simulink model "TDPBehaviourSim"  (R2020b)
settings: Solver=VariableStepAuto  StartTime=0.0  StopTime=200  FixedStep=sampleTime  RelTol=1e-3  EnableMultiTasking=on
values from neighbouring files (symbols this model uses):
  angThresh = pi/16    (= 0.196349540849)    [GameParameters.m]
  attackerKickSpeed = 0.3    [GameParameters.m]
  AwayFormation1 = [9.5 4 pi ... (first row only)    [FormationPoses.m]    (also in GameParameters.m)
  ballAngleNoise = pi/24    (= 0.1308996939)    [GameParameters.m]
  ballThresh = playerRadius + 0.03    (= 0.11)    [GameParameters.m]
  ballVelNoise = 0.05    [GameParameters.m]
  distThresh = 0.1    [GameParameters.m]
  fieldCenter = [mean(fieldLimitsX) mean(fieldLimitsY)]    [GameParameters.m]
  fieldLimitsX = [1 10]    [GameParameters.m]
  fieldLimitsY = [1 7]    [GameParameters.m]
  goalPosts = [1  2.7 2 ... (first row only)    [GameParameters.m]
  HomeFormation1 = [1.5 4 0 ... (first row only)    [FormationPoses.m]    (also in GameParameters.m)
  maxSpeed = 0.1    [GameParameters.m]
  maxTurnSpeed = 0.05    [GameParameters.m]
  playerRadius = 0.08    [GameParameters.m]
  sampleTime = 0.5    [GameParameters.m]
undefined symbols (not defined in the file or in its folder): DiscIntNeverNeededParam
libraries: mobileRoboticsLib x33, soccerRobotLib x16
(part 2 of 2)

== system TDPBehaviourSim/Home Team/GK Information for Decision Making ==
  In1 : Inport
  In2 : Inport  Port=2
  Personal Information : BusSelector  OutputSignals=Home Team GK pos,Home Team GK obj,Home Team GK robot,Home GK Velocity
  TeamMatePositions : BusSelector  OutputSignals=Home Team Defender pos,Home Team MidFielder pos,Home Team Striker pos
  <Home Team GK pos> : Outport
  <Home Team GK obj> : Outport  Port=2
  <Home Team GK robot> : Outport  Port=3
  <Home GK Velocity> : Outport  Port=4
  <Home Team Defender pos> : Outport  Port=5
  <Home Team MidFielder pos> : Outport  Port=6
  <Home Team Striker pos> : Outport  Port=7
  wires:
  Personal Information/2 -> <Home Team GK obj>/1  "<Home Team GK obj>"
  Personal Information/4 -> <Home GK Velocity>/1  "<Home GK Velocity>"
  TeamMatePositions/3 -> <Home Team Striker pos>/1  "<Home Team Striker pos>"
  In1/1 -> Personal Information/1
  In2/1 -> TeamMatePositions/1
  Personal Information/1 -> <Home Team GK pos>/1  "<Home Team GK pos>"
  TeamMatePositions/1 -> <Home Team Defender pos>/1  "<Home Team Defender pos>"
  Personal Information/3 -> <Home Team GK robot>/1  "<Home Team GK robot>"
  TeamMatePositions/2 -> <Home Team MidFielder pos>/1  "<Home Team MidFielder pos>"

== system TDPBehaviourSim/Home Team/MidFielder Information For Decision Making ==
  In1 : Inport
  In2 : Inport  Port=2
  Bus Selector : BusSelector  OutputSignals=Home Team Midfielder obj,Home Team Midfielder robot,Home Team MidFielder pos,Home Mid Vel
  Bus Selector1 : BusSelector  OutputSignals=Home Team Striker pos,Home Team Defender pos,Home Team GK pos
  <Home Team Midfielder obj> : Outport
  <Home Team Midfielder robot> : Outport  Port=2
  <Home Team MidFielder pos> : Outport  Port=3
  <Home Mid Vel> : Outport  Port=4
  <Home Team Striker pos> : Outport  Port=5
  <Home Team Defender pos> : Outport  Port=6
  <Home Team GK pos> : Outport  Port=7
  wires:
  Bus Selector1/3 -> <Home Team GK pos>/1  "<Home Team GK pos>"
  Bus Selector1/1 -> <Home Team Striker pos>/1  "<Home Team Striker pos>"
  Bus Selector/1 -> <Home Team Midfielder obj>/1  "<Home Team Midfielder obj>"
  In2/1 -> Bus Selector/1
  In1/1 -> Bus Selector1/1
  Bus Selector1/2 -> <Home Team Defender pos>/1  "<Home Team Defender pos>"
  Bus Selector/2 -> <Home Team Midfielder robot>/1  "<Home Team Midfielder robot>"
  Bus Selector/3 -> <Home Team MidFielder pos>/1  "<Home Team MidFielder pos>"
  Bus Selector/4 -> <Home Mid Vel>/1  "<Home Mid Vel>"

== system TDPBehaviourSim/Home Team/Striker Information fot Decision Making ==
  In1 : Inport
  In2 : Inport  Port=2
  Bus Selector : BusSelector  OutputSignals=Home Team Striker robot,Home Team Striker obj,Home Team Striker pos,Home Striker Vel
  Bus Selector1 : BusSelector  OutputSignals=Home Team GK pos,Home Team Defender pos,Home Team MidFielder pos
  <Home Team Striker robot> : Outport
  <Home Team Striker obj> : Outport  Port=2
  <Home Team Striker pos> : Outport  Port=3
  <Home Striker Vel> : Outport  Port=4
  <Home Team GK pos> : Outport  Port=5
  <Home Team Defender pos> : Outport  Port=6
  <Home Team MidFielder pos> : Outport  Port=7
  wires:
  Bus Selector1/1 -> <Home Team GK pos>/1  "<Home Team GK pos>"
  In1/1 -> Bus Selector/1
  In2/1 -> Bus Selector1/1
  Bus Selector/1 -> <Home Team Striker robot>/1  "<Home Team Striker robot>"
  Bus Selector/4 -> <Home Striker Vel>/1  "<Home Striker Vel>"
  Bus Selector/2 -> <Home Team Striker obj>/1  "<Home Team Striker obj>"
  Bus Selector/3 -> <Home Team Striker pos>/1  "<Home Team Striker pos>"
  Bus Selector1/3 -> <Home Team MidFielder pos>/1  "<Home Team MidFielder pos>"
  Bus Selector1/2 -> <Home Team Defender pos>/1  "<Home Team Defender pos>"

== stateflow chart TDPBehaviourSim/Away Team/Chart ==
  state Information
    en,du:
    position;
    players;
    objects
    nextVelocity = [velocity(1); velocity(2); velocity(3)];
    [objSeen,objDIst,objAng] = detectObj(objects,1);
    toObj = [objSeen,objDIst,objAng];
    teammates;
  (default) -> Information
  data: position input; velocity input size=[3 1]; nextVelocity output =[0;0;0]; players input; teammates input; objects input; objAng local; objDIst local; objSeen local; toObj output

== stateflow chart TDPBehaviourSim/Away Team/Chart1 ==
  state Information
    en,du:
    position;
    nextVelocity = [velocity(1); velocity(2); velocity(3)];
    [objSeen,objDIst,objAng] = detectObj(objects,1);
    toObj = [objSeen,objDIst,objAng];
    teammates;
    players;
    objects;
  (default) -> Information
  data: position input; velocity input size=[3 1]; nextVelocity output =[0;0;0]; players input; teammates input; objects input; toObj output; objAng local; objDIst local; objSeen local

== stateflow chart TDPBehaviourSim/Away Team/Chart2 ==
  state Information
    en,du:
    position;
    nextVelocity = [velocity(1);velocity(2);velocity(3)]
    teammates;
    players;
    [objSeen,objDIst,objAng] = detectObj(objects,1);
    toObj = [objSeen,objDIst,objAng];
    objects
  (default) -> Information
  data: position input; velocity input size=[3 1]; nextVelocity output =[0;0;0]; players input; teammates input; objects input; toObj output; objAng local; objDIst local; objSeen local

== stateflow chart TDPBehaviourSim/Away Team/Chart3 ==
  state Information
    en,du:
    position;
    nextVelocity = [velocity(1);velocity(2);velocity(3)];
    teammates;
    objects;
    players;
    [objSeen,objDIst,objAng] = detectObj(objects,1);
    toObj = [objSeen,objDIst,objAng];
  (default) -> Information
  data: position input; velocity input size=[3 1]; nextVelocity output =[0;0;0]; players input; teammates input; objects input; toObj output; objAng local; objDIst local; objSeen local

== stateflow chart TDPBehaviourSim/GameState ==
  state BallDynamics [parallel]
    en:
    setBallState(fieldCenter,0,0);
    settings: executionOrder=2
    state InBounds
      en:
      randNum = randn(1,2);
      du:
      gamestate.state = getGameState;
      state BallFree
      state BallHeld
        en,du:
        ballPose = [robo_pos(3*holder_idx-2) robo_pos(3*holder_idx-1)] + ...
        (playerRadius+ballThresh)*[cos(robo_pos(3*holder_idx)) sin(robo_pos(3*holder_idx))];
      (default) -> BallFree
      BallHeld -> BallFree : after(1,sec)[ballKicked==1]{setBallState(ballPose,ballVel + ballVelNoise,robo_pos(3*holder_idx))}
      BallFree -> BallHeld : [gamestate.possession(1)~=0]
    state OutOfBounds
      en,du:
      gamestate.state = getGameState;
      setBallState(ballPose,0,0);
      if lastPossession == 1
      end
    state CornerOrGOakKick
      en,du:
      gamestate.state = getGameState;
    state GoalScored
      en,du:
      gamestate.state = getGameState;
    (default) -> InBounds
    OutOfBounds -> InBounds : [gamestate.state==gameSituation(1)]
    InBounds -> OutOfBounds [order 1] : [gamestate.state == gameSituation(2)]
    GoalScored -> InBounds : [gamestate.state==gameSituation(1)]
    InBounds -> GoalScored [order 2] : [gamestate.state==gameSituation(3)]
    CornerOrGOakKick -> InBounds : [gamestate.state==gameSituation(1)]
    InBounds -> CornerOrGOakKick [order 3] : [gamestate.state==gameSituation(4)]
  state TimeSetter [parallel]
    en,du:
    settings: executionOrder=3
    state EarlyGame
      en,du:
      time=elapsed(sec);
      gamestate.time=gameTime(1);
    state MidGame
      en,du:
      time=elapsed(sec);
      gamestate.time=gameTime(2);
    state LateGame
      en,du:
      time=elapsed(sec);
      gamestate.time=gameTime(3)
    state GameOver
      en:
      done = 1;
    (default) -> EarlyGame
    EarlyGame -> MidGame : [time==400]
    MidGame -> LateGame : [time==800]
    LateGame -> GameOver : [time==1200]
  state state = getGameState [function]
    note: Returns the game state depending on the position of the ball on the field
    (default) -> (junction 52)
    (junction 52) -> (junction 53) [order 1] : [ballPose(1) <= fieldLimitsX(1) || ballPose(1) >= fieldLimitsX(2) || ...
        |  ballPose(2) <= fieldLimitsY(1) || ballPose(2) >= fieldLimitsY(2)]
    (junction 52) -> (junction 56) [order 2] : {state = gameSituation.InPlay;}
    (junction 53) -> (junction 54)
    (junction 54) -> (junction 55) [order 1] : [ballPose(2)<=goalPosts(1,2) && ...
        | ballPose(2) >= goalPosts(2,2)]
    (junction 54) -> (junction 57) [order 2] : {state = gameSituation.OutOfPlay;}
    (junction 55) -> (junction 58) : {state = gameSituation.GoalScored;}
    (junction 57) -> (junction 56)
    (junction 58) -> (junction 57)
  state setBallState(pos,vel,theta) [function]
  state DeterminePossession [parallel]
    en,du:
    gamestate.possession = [holded,holder_idx];
    if gamestate.possession(2)>0 &&gamestate.possession(2)<=4
    gamestate.possessingTeam = 1;
    lastPossession = 1;
    elseif gamestate.possession(2)>=5
    gamestate.possessingTeam = 2;
    lastPossession = 2;
    else
    gamestate.possessingTeam = 0;
    end
    settings: executionOrder=1
  data: sf_internal_action_state_placeholder_data local double size=1 =0; state function_output; pos function_input double size=[1 2]; vel function_input double size=1; theta function_input double size=1; ballPose output =fieldCenter; attackerKickSpeed parameter; ballThresh parameter; ballDist local; playerRadius parameter double; fieldLimitsX parameter; fieldLimitsY parameter; goalPosts parameter; fieldCenter parameter; robo_pos input; gamestate output Bus: gameSituationBus; ballVel local =0.5; ballVelNoise parameter; ballAngleNoise parameter; randNum local =[0 0]; ballKicked local =0; time local; done output =0; lastPossession local =0; holded input; holder_idx input

== stateflow chart TDPBehaviourSim/TeamActivityAssignment ==
  state SetTeamActivity [parallel]
    en,du:
    settings: executionOrder=1
    state InPlay
      state Attack
        en,du:
        homeTeam.inPossession = 1;
        homeTeam.activity = teamAction(1);
        homeTeam.ballHolder = gamestate.possession(2);
        awayTeam.inPossession = 0;
        awayTeam.activity = teamAction(2);
        awayTeam.ballHolder = 0;
      state Defend
        en,du:
        homeTeam.inPossession = 0;
        homeTeam.activity = teamAction(1);
        homeTeam.ballHolder = gamestate.possession(2);
        awayTeam.inPossession = 1;
        awayTeam.activity = teamAction(2);
        awayTeam.ballHolder = 0;
      state CaptureBall
        en,du:
        homeTeam.inPossession = 0;
        homeTeam.ballHolder = 0;
        awayTeam.inPossession = 0;
        awayTeam.ballHolder = 0;
        homeTeam.activity = teamAction(3);
        awayTeam.activity = teamAction(3);
      (default) -> (junction 7)
      (junction 25) -> Attack
      (junction 26) -> (junction 25) : [gamestate.possessingTeam==1]
      (junction 7) -> Attack [order 1] : [gamestate.possessingTeam == 1]
      (junction 7) -> (junction 10) [order 2]
      Attack -> (junction 23) [order 2]
      (junction 23) -> (junction 24) : [gamestate.possessingTeam==0]
      Attack -> Defend [order 1] : [gamestate.possessingTeam==2]
      Defend -> Attack [order 1] : [gamestate.possessingTeam==1]
      (junction 10) -> Defend [order 1] : [gamestate.possessingTeam==2]
      (junction 10) -> (junction 14) [order 2]
      Defend -> CaptureBall [order 2] : [gamestate.possessingTeam==0]
      CaptureBall -> Defend [order 1] : [gamestate.possessingTeam==2]
      (junction 14) -> CaptureBall
      (junction 24) -> CaptureBall
      CaptureBall -> (junction 26) [order 2]
    state OutOfPlay
    state GoalScored
    state GoalCornerKick
    (default) -> (junction 35)
    GoalCornerKick -> InPlay : [gamestate.state==gameSituation(1)]
    (junction 35) -> InPlay [order 1]
    (junction 35) -> (junction 39) [order 2]
    InPlay -> GoalScored [order 3] : [gamestate.state==gameSituation(3)]
    InPlay -> GoalCornerKick [order 2] : [gamestate.state==gameSituation(4)]
    InPlay -> OutOfPlay [order 1] : [gamestate.state==gameSituation(2)]
    OutOfPlay -> InPlay : [gamestate.state==gameSituation(1)]
    (junction 39) -> OutOfPlay [order 1] : [gamestate.state==gameSituation(2)]
    (junction 39) -> (junction 43) [order 2]
    (junction 43) -> GoalScored [order 1] : [gamestate.state==gameSituation(3)]
    (junction 43) -> (junction 47) [order 2]
    (junction 47) -> GoalCornerKick : [gamestate.state==gameSituation(4)]
  data: gamestate input Bus: gameSituationBus; homeTeam output Bus: teamActivity; awayTeam output Bus: teamActivity

== matlab function TDPBehaviourSim/MATLAB Function ==
  data: home input; holded output; away input; indexholder output
function [holded,indexholder]=findholder(home,away)
holded=false;
holdingTeam= 0;
indexholder=0;
awayHolds=0;
homeHolds=0;
determineholder=0;
%% This function returns if ball is holded or not and the player's index if holded
homeindexholder = find(home(:,1) ~= 0 & home(:,2) < 0.3  & home(:,2) > 0  & home(:,3) > -pi/4 & home(:,3) < pi/4);
awayindexholder = find(away(:,1) ~= 0 & away(:,2) < 0.3 & away(:,2) > 0 & away(:,3) >-pi/4  & away(:,3) < pi/4);
awayHolds = ~isempty(awayindexholder);
homeHolds = ~isempty(homeindexholder);

if awayHolds || homeHolds
    holded = true;
    if homeHolds && ~awayHolds
        if size(homeindexholder,1)== 1
            indexholder = homeindexholder(1);
        else
            indexholder = homeindexholder(randi([1,size(homeindexholder,1)]));            
        end
    elseif awayHolds && ~homeHolds
        if size(homeindexholder,1)>1
            indexholder = awayindexholder(randi([1,size(awayindexholder,1)])) + 4;
        else
            indexholder = awayindexholder(1);
        end
    elseif  homeHolds && awayHolds
        determineholder = [homeindexholder;awayindexholder+4];
        indexholder = determineholder(randi([1,size(determineholder,1)]));
    end
    
end
end

== stateflow chart TDPBehaviourSim/Home Team/Chart4 ==
  state [vel,done] = goToPose(goal) [function]
    note: Tracks a position. Once reached, the robot will turn in place until a reference angle is met.
    (default) -> (junction 225) : {
        | vel = [0;0;0];
        | [goalDist,goalAng] = calcBearing(goal(1:2));
        | trackAng = angdiff(position(3),goal(3));
        | }
    (junction 225) -> (junction 226) [order 1] : % Track the position if outside the distance threshold
        | [goalDist > distThresh]
    (junction 225) -> (junction 227) [order 2] : % Else, turn in place until the angular reference is met
    (junction 226) -> (junction 234) : {vel = trackDetection(goalDist,goalAng);}
    (junction 227) -> (junction 228) [order 1] : [trackAng > angThresh]
    (junction 227) -> (junction 229) [order 2]
    (junction 228) -> (junction 233) : {vel(3) = 1;}
    (junction 229) -> (junction 230) [order 1] : [trackAng < -angThresh]
    (junction 229) -> (junction 231) [order 2]
    (junction 230) -> (junction 232) : {vel(3) = -1;}
    (junction 232) -> (junction 231)
    (junction 233) -> (junction 232)
    (junction 234) -> (junction 233)
    (junction 231) -> (junction 235) : {done = (goalDist <= distThresh) && (abs(trackAng) <= angThresh);}
  state PlayerMovement [parallel]
    en:
    nextVelocity = velocity;
    du:
    settings: executionOrder=1
    state InPlay
      state Attack
        state BallHolder
          en,du:
          nextVelocity = goToPose([1,4,0]);
        state OtherTeammateBallHolder
          en,du:
          nextVelocity=goToPose([8,3,0]);
        (default) -> (junction 338)
        (junction 338) -> BallHolder [order 1]
        (junction 338) -> (junction 339) [order 2]
        (junction 339) -> OtherTeammateBallHolder : [homeTeam.ballHolder~=robotIndex]
      state Defend
      state GetBall
        state LookForBall
          en,du:
          nextVelocity = [0;0;-1];
        state GoToBall
          en,du:
          nextVelocity= trackDetection(ballDist,ballAng);
        (default) -> LookForBall
        LookForBall -> GoToBall : after(1,sec)[ballSeen&&ballDist<2.5&&ballAng<angThresh&&ballAng<-angThresh]
        GoToBall -> LookForBall : [~ballSeen]
      (default) -> (junction 315)
      Attack -> (junction 314) [order 1]
      (junction 314) -> (junction 319) : [homeTeam.activity==teamAction(3)]
      (junction 315) -> Attack [order 1] : [homeTeam.activity == teamAction(1)]
      (junction 316) -> Attack
      (junction 315) -> (junction 317) [order 2]
      (junction 318) -> (junction 316) : [homeTeam.activity==teamAction(1)]
      Attack -> Defend [order 2] : [homeTeam.activity==teamAction(2)]
      Defend -> Attack [order 1] : [homeTeam.activity==teamAction(1)]
      (junction 317) -> Defend [order 1] : [homeTeam.activity == teamAction(2)]
      (junction 317) -> (junction 320) [order 2]
      Defend -> GetBall [order 2] : [homeTeam.activity==teamAction(3)]
      GetBall -> Defend [order 2] : [homeTeam.activity==teamAction(2)]
      GetBall -> (junction 318) [order 1]
      (junction 319) -> GetBall
      (junction 320) -> GetBall
    (default) -> InPlay
  state Finder [parallel]
    settings: executionOrder=2
    state F [parallel]
      en,du:
      [ballSeen,ballDist,ballAng] = detectObj(objects,1);
      toBall = [ballSeen,ballDist,ballAng];
      settings: executionOrder=1
  state [dist,ang] = calcBearing(goal) [function]
    (default) -> (junction 219) : % Calculate distance and angle to location
        | {
        | err = goal(1:2) - [position(1) position(2)];
        | dist = norm(err);
        | ang = angdiff(position(3),atan2(err(2),err(1)));
        | }
  state [vel,done] = turnToPoint(goal) [function]
    note: Tracks a position. Once reached, the robot will turn in place until a reference angle is met.
    (default) -> (junction 255) : % Turn in place until the angular reference is met
        | {
        | done = false;
        | vel = [0;0;0];
        | [goalDist,goalAng] = calcBearing(goal(1:2));
        | }
    (junction 255) -> (junction 256) [order 1] : [goalAng > angThresh]
    (junction 255) -> (junction 257) [order 2]
    (junction 256) -> (junction 261) : {vel(3) = 1;}
    (junction 257) -> (junction 258) [order 1] : [goalAng < -angThresh]
    (junction 257) -> (junction 259) [order 2] : {done = true;}
    (junction 258) -> (junction 260) : {vel(3) = -1;}
    (junction 260) -> (junction 259)
    (junction 261) -> (junction 260)
  state vel = trackDetection(dist,ang) [function]
    note: Uses range and bearing to track an object
    (default) -> (junction 277) : {
        | vel = [0;0;0];
        | }
    (junction 277) -> (junction 276) [order 1] : % Turn in place
        | % if no detection
        | [dist < 0]
    (junction 276) -> (junction 286) : {vel(3) = 1;}
    (junction 277) -> (junction 278) [order 2]
    (junction 278) -> (junction 279) [order 1] : % Forward speed
        | [dist > distThresh]
    (junction 279) -> (junction 281) : {vel(1) = maxSpeed;}
    (junction 278) -> (junction 280) [order 2]
    (junction 281) -> (junction 280)
    (junction 280) -> (junction 282)
    (junction 282) -> (junction 283) [order 1] : % Turning speed
        | [ang > angThresh]
    (junction 283) -> (junction 289) : {vel(3) = maxTurnSpeed;}
    (junction 282) -> (junction 284) [order 2]
    (junction 284) -> (junction 285) [order 1] : [ang < -angThresh]
    (junction 284) -> (junction 287) [order 2]
    (junction 285) -> (junction 288) : {vel(3) = -1;}
    (junction 286) -> (junction 287)
    (junction 288) -> (junction 287)
    (junction 289) -> (junction 288)
  data: vel function_output; done function_output; goal function_input; goal function_input; dist function_output; ang function_output; goal function_input; vel function_output; done function_output; dist function_input; ang function_input; vel function_output; homeTeam input; position input; velocity input; nextVelocity output =[0;0;0.1]; players input; teammates input; objects input; angThresh parameter; distThresh parameter; maxSpeed parameter; maxTurnSpeed parameter; robotIndex local =3; ballAng local; ballDist local; ballSeen local; toBall output

== matlab function TDPBehaviourSim/Game Visualiser/Plot Soccer Field ==
function plotSoccerField
% Plots the soccer field once the figure window for the environment has
% been initialized

coder.extrinsic('evalin');
persistent hasPlotted
if isempty(hasPlotted)
    evalin('base','plotSoccerField');
    hasPlotted = true;
end

== matlab function TDPBehaviourSim/Game Visualiser/Subsystem/Object Matrix Creator ==
  data: BallPos input; objectPositions output; goalPosts input
function objectPositions = SetPositions(BallPos,goalPosts)

objectPositions =[BallPos(1) BallPos(2) 1;goalPosts];

== stateflow chart TDPBehaviourSim/Home Team/Chart ==
  state PlayerMovement [parallel]
    en:
    nextVelocity = velocity;
    du:
    settings: executionOrder=2
    state InPlay
      state Attack
        state BallHolder
        state OtherTeammateBallHolder
        (default) -> (junction 256)
        (junction 256) -> BallHolder [order 1]
        (junction 256) -> (junction 257) [order 2]
        OtherTeammateBallHolder -> BallHolder : [homeTeam.ballHolder==robotIndex]
        BallHolder -> OtherTeammateBallHolder : [homeTeam.ballHolder~=robotIndex]
        (junction 257) -> OtherTeammateBallHolder : [homeTeam.ballHolder~=robotIndex]
      state Defend
      state GetBall
      (default) -> (junction 233)
      Attack -> (junction 232) [order 1]
      (junction 233) -> Attack [order 1] : [homeTeam.activity == teamAction(1)]
      (junction 232) -> (junction 237) : [homeTeam.activity==teamAction(3)]
      (junction 233) -> (junction 235) [order 2]
      (junction 234) -> Attack
      (junction 236) -> (junction 234) : [homeTeam.activity==teamAction(1)]
      Attack -> Defend [order 2] : [homeTeam.activity==teamAction(2)]
      Defend -> Attack [order 1] : [homeTeam.activity==teamAction(1)]
      (junction 235) -> Defend [order 1] : [homeTeam.activity == teamAction(2)]
      (junction 235) -> (junction 238) [order 2]
      Defend -> GetBall [order 2] : [homeTeam.activity==teamAction(3)]
      GetBall -> Defend [order 2] : [homeTeam.activity==teamAction(2)]
      GetBall -> (junction 236) [order 1]
      (junction 237) -> GetBall
      (junction 238) -> GetBall
    (default) -> InPlay
  state PlayerDistances [parallel]
    settings: executionOrder=1
    state FindObject
      en,du:
      [objSeen,objDist,objAng] = detectObj(objects,obj);
      toObj = [objSeen,objDist,objAng];
    (default) -> FindObject
  state [vel,done] = goToPose(goal) [function]
    note: Tracks a position. Once reached, the robot will turn in place until a reference angle is met.
    (default) -> (junction 138) : {
        | vel = [0;0;0];
        | [goalDist,goalAng] = calcBearing(goal(1:2));
        | trackAng = angdiff(position(3),goal(3));
        | }
    (junction 138) -> (junction 139) [order 1] : % Track the position if outside the distance threshold
        | [goalDist > distThresh]
    (junction 138) -> (junction 140) [order 2] : % Else, turn in place until the angular reference is met
    (junction 139) -> (junction 147) : {vel = trackDetection(goalDist,goalAng);}
    (junction 140) -> (junction 141) [order 1] : [trackAng > angThresh]
    (junction 140) -> (junction 142) [order 2]
    (junction 141) -> (junction 146) : {vel(3) = 1;}
    (junction 142) -> (junction 143) [order 1] : [trackAng < -angThresh]
    (junction 142) -> (junction 144) [order 2]
    (junction 143) -> (junction 145) : {vel(3) = -1;}
    (junction 145) -> (junction 144)
    (junction 146) -> (junction 145)
    (junction 147) -> (junction 146)
    (junction 144) -> (junction 148) : {done = (goalDist <= distThresh) && (abs(trackAng) <= angThresh);}
  state [dist,ang] = calcBearing(goal) [function]
    (default) -> (junction 168) : % Calculate distance and angle to location
        | {
        | err = goal(1:2) - [position(1) position(2)];
        | dist = norm(err);
        | ang = angdiff(position(3),atan2(err(2),err(1)));
        | }
  state [vel,done] = turnToPoint(goal) [function]
    note: Tracks a position. Once reached, the robot will turn in place until a reference angle is met.
    (default) -> (junction 117) : % Turn in place until the angular reference is met
        | {
        | done = false;
        | vel = [0;0;0];
        | [goalDist,goalAng] = calcBearing(goal(1:2));
        | }
    (junction 117) -> (junction 118) [order 1] : [goalAng > angThresh]
    (junction 117) -> (junction 119) [order 2]
    (junction 118) -> (junction 123) : {vel(3) = 1;}
    (junction 119) -> (junction 120) [order 1] : [goalAng < -angThresh]
    (junction 119) -> (junction 121) [order 2] : {done = true;}
    (junction 120) -> (junction 122) : {vel(3) = -1;}
    (junction 122) -> (junction 121)
    (junction 123) -> (junction 122)
  state vel = trackDetection(dist,ang) [function]
    note: Uses range and bearing to track an object
    (default) -> (junction 79) : {
        | vel = [0;0;0];
        | }
    (junction 79) -> (junction 78) [order 1] : % Turn in place
        | % if no detection
        | [dist < 0]
    (junction 78) -> (junction 88) : {vel(3) = 1;}
    (junction 79) -> (junction 80) [order 2]
    (junction 80) -> (junction 81) [order 1] : % Forward speed
        | [dist > distThresh]
    (junction 81) -> (junction 83) : {vel(1) = maxSpeed;}
    (junction 80) -> (junction 82) [order 2]
    (junction 83) -> (junction 82)
    (junction 82) -> (junction 84)
    (junction 84) -> (junction 85) [order 1] : % Turning speed
        | [ang > angThresh]
    (junction 85) -> (junction 91) : {vel(3) = maxTurnSpeed;}
    (junction 84) -> (junction 86) [order 2]
    (junction 86) -> (junction 87) [order 1] : [ang < -angThresh]
    (junction 86) -> (junction 89) [order 2]
    (junction 87) -> (junction 90) : {vel(3) = -1;}
    (junction 88) -> (junction 89)
    (junction 90) -> (junction 89)
    (junction 91) -> (junction 90)
  data: vel function_output; done function_output; goal function_input; goal function_input; dist function_output; ang function_output; goal function_input; vel function_output; done function_output; dist function_input; ang function_input; vel function_output; homeTeam input Bus: teamActivity; position input; velocity input double; nextVelocity output; players input; teammates input; objects input; y local; z local; objDist local; objAng local; objSeen local; plDist local; plSeen local; plAng local; distThresh parameter; angThresh parameter; x local; maxSpeed parameter; maxTurnSpeed parameter; obj local =1; toObj output; robotIndex local =1

== stateflow chart TDPBehaviourSim/Home Team/Chart1 ==
  state [vel,done] = goToPose(goal) [function]
    note: Tracks a position. Once reached, the robot will turn in place until a reference angle is met.
    (default) -> (junction 225) : {
        | vel = [0;0;0];
        | [goalDist,goalAng] = calcBearing(goal(1:2));
        | trackAng = angdiff(position(3),goal(3));
        | }
    (junction 225) -> (junction 226) [order 1] : % Track the position if outside the distance threshold
        | [goalDist > distThresh]
    (junction 225) -> (junction 227) [order 2] : % Else, turn in place until the angular reference is met
    (junction 226) -> (junction 234) : {vel = trackDetection(goalDist,goalAng);}
    (junction 227) -> (junction 228) [order 1] : [trackAng > angThresh]
    (junction 227) -> (junction 229) [order 2]
    (junction 228) -> (junction 233) : {vel(3) = 1;}
    (junction 229) -> (junction 230) [order 1] : [trackAng < -angThresh]
    (junction 229) -> (junction 231) [order 2]
    (junction 230) -> (junction 232) : {vel(3) = -1;}
    (junction 232) -> (junction 231)
    (junction 233) -> (junction 232)
    (junction 234) -> (junction 233)
    (junction 231) -> (junction 235) : {done = (goalDist <= distThresh) && (abs(trackAng) <= angThresh);}
  state PlayerMovement [parallel]
    en:
    nextVelocity = velocity;
    du:
    settings: executionOrder=1
    state InPlay
      state Attack
        en,du:
        state BallHolder
          en,du:
          nextVelocity = goToPose([8,4,0]);
        state OtherTeammateBallHolder
          en,du:
          nextVelocity = goToPose([3,4,0]);
        (default) -> (junction 348)
        (junction 348) -> BallHolder [order 1]
        (junction 348) -> (junction 351) [order 2]
        (junction 351) -> OtherTeammateBallHolder : [homeTeam.ballHolder~=robotIndex]
      state Defend
      state GetBall
        state LookForBall
          en,du:
          nextVelocity = [0;0;-1];
        state GoToBall
          en,du:
          nextVelocity= trackDetection(ballDist,ballAng);
        (default) -> LookForBall
        LookForBall -> GoToBall : after(1,sec)[ballSeen&&ballDist<2.5&&ballAng<angThresh&&ballAng<-angThresh]
        GoToBall -> LookForBall : [~ballSeen]
      (default) -> (junction 317)
      Attack -> (junction 328) [order 1]
      (junction 328) -> (junction 331) : [homeTeam.activity==teamAction(3)]
      (junction 317) -> Attack [order 1] : [homeTeam.activity == teamAction(1)]
      (junction 327) -> Attack
      (junction 317) -> (junction 318) [order 2]
      (junction 330) -> (junction 327) : [homeTeam.activity==teamAction(1)]
      Attack -> Defend [order 2] : [homeTeam.activity==teamAction(2)]
      Defend -> Attack [order 1] : [homeTeam.activity==teamAction(1)]
      (junction 318) -> Defend [order 1] : [homeTeam.activity == teamAction(2)]
      (junction 318) -> (junction 319) [order 2]
      Defend -> GetBall [order 2] : [homeTeam.activity==teamAction(3)]
      GetBall -> Defend [order 2] : [homeTeam.activity==teamAction(2)]
      GetBall -> (junction 330) [order 1]
      (junction 331) -> GetBall
      (junction 319) -> GetBall
    (default) -> InPlay
  state PlayerDistances [parallel]
    settings: executionOrder=2
    state FindObject [parallel]
      en,du:
      [ballSeen,ballDist,ballAng] = detectObj(objects,1);
      toBall = [ballSeen,ballDist,ballAng];
      settings: executionOrder=1
  state [dist,ang] = calcBearing(goal) [function]
    (default) -> (junction 219) : % Calculate distance and angle to location
        | {
        | err = goal(1:2) - [position(1) position(2)];
        | dist = norm(err);
        | ang = angdiff(position(3),atan2(err(2),err(1)));
        | }
  state [vel,done] = turnToPoint(goal) [function]
    note: Tracks a position. Once reached, the robot will turn in place until a reference angle is met.
    (default) -> (junction 255) : % Turn in place until the angular reference is met
        | {
        | done = false;
        | vel = [0;0;0];
        | [goalDist,goalAng] = calcBearing(goal(1:2));
        | }
    (junction 255) -> (junction 256) [order 1] : [goalAng > angThresh]
    (junction 255) -> (junction 257) [order 2]
    (junction 256) -> (junction 261) : {vel(3) = 1;}
    (junction 257) -> (junction 258) [order 1] : [goalAng < -angThresh]
    (junction 257) -> (junction 259) [order 2] : {done = true;}
    (junction 258) -> (junction 260) : {vel(3) = -1;}
    (junction 260) -> (junction 259)
    (junction 261) -> (junction 260)
  state vel = trackDetection(dist,ang) [function]
    note: Uses range and bearing to track an object
    (default) -> (junction 277) : {
        | vel = [0;0;0];
        | }
    (junction 277) -> (junction 276) [order 1] : % Turn in place
        | % if no detection
        | [dist < 0]
    (junction 276) -> (junction 286) : {vel(3) = 1;}
    (junction 277) -> (junction 278) [order 2]
    (junction 278) -> (junction 279) [order 1] : % Forward speed
        | [dist > distThresh]
    (junction 279) -> (junction 281) : {vel(1) = maxSpeed;}
    (junction 278) -> (junction 280) [order 2]
    (junction 281) -> (junction 280)
    (junction 280) -> (junction 282)
    (junction 282) -> (junction 283) [order 1] : % Turning speed
        | [ang > angThresh]
    (junction 283) -> (junction 289) : {vel(3) = maxTurnSpeed;}
    (junction 282) -> (junction 284) [order 2]
    (junction 284) -> (junction 285) [order 1] : [ang < -angThresh]
    (junction 284) -> (junction 287) [order 2]
    (junction 285) -> (junction 288) : {vel(3) = -1;}
    (junction 286) -> (junction 287)
    (junction 288) -> (junction 287)
    (junction 289) -> (junction 288)
  data: vel function_output; done function_output; goal function_input; goal function_input; dist function_output; ang function_output; goal function_input; vel function_output; done function_output; dist function_input; ang function_input; vel function_output; homeTeam input; position input; velocity input; nextVelocity output =[0;0;0]; players input; teammates input; objects input; objAng local; angThresh parameter; distThresh parameter; maxSpeed parameter; maxTurnSpeed parameter; robotIndex local =2; ballAng local; ballDist local; ballSeen local; toBall output

== stateflow chart TDPBehaviourSim/Home Team/Chart2 ==
  state [vel,done] = goToPose(goal) [function]
    note: Tracks a position. Once reached, the robot will turn in place until a reference angle is met.
    (default) -> (junction 225) : {
        | vel = [0;0;0];
        | [goalDist,goalAng] = calcBearing(goal(1:2));
        | trackAng = angdiff(position(3),goal(3));
        | }
    (junction 225) -> (junction 226) [order 1] : % Track the position if outside the distance threshold
        | [goalDist > distThresh]
    (junction 225) -> (junction 227) [order 2] : % Else, turn in place until the angular reference is met
    (junction 226) -> (junction 234) : {vel = trackDetection(goalDist,goalAng);}
    (junction 227) -> (junction 228) [order 1] : [trackAng > angThresh]
    (junction 227) -> (junction 229) [order 2]
    (junction 228) -> (junction 233) : {vel(3) = 1;}
    (junction 229) -> (junction 230) [order 1] : [trackAng < -angThresh]
    (junction 229) -> (junction 231) [order 2]
    (junction 230) -> (junction 232) : {vel(3) = -1;}
    (junction 232) -> (junction 231)
    (junction 233) -> (junction 232)
    (junction 234) -> (junction 233)
    (junction 231) -> (junction 235) : {done = (goalDist <= distThresh) && (abs(trackAng) <= angThresh);}
  state PlayerMovement [parallel]
    en:
    nextVelocity = velocity;
    du:
    settings: executionOrder=1
    state InPlay
      state Attack
        state BallHolder
        state OtherTeammateBallHolder
        (default) -> (junction 339)
        (junction 339) -> BallHolder [order 1]
        (junction 339) -> (junction 340) [order 2]
        (junction 340) -> OtherTeammateBallHolder : [homeTeam.ballHolder~=robotIndex]
      state Defend
      state GetBall
      (default) -> (junction 316)
      Attack -> (junction 315) [order 1]
      (junction 315) -> (junction 320) : [homeTeam.activity==teamAction(3)]
      (junction 316) -> Attack [order 1] : [homeTeam.activity == teamAction(1)]
      (junction 317) -> Attack
      (junction 316) -> (junction 318) [order 2]
      (junction 319) -> (junction 317) : [homeTeam.activity==teamAction(1)]
      Attack -> Defend [order 2] : [homeTeam.activity==teamAction(2)]
      Defend -> Attack [order 1] : [homeTeam.activity==teamAction(1)]
      (junction 318) -> Defend [order 1] : [homeTeam.activity == teamAction(2)]
      (junction 318) -> (junction 321) [order 2]
      Defend -> GetBall [order 2] : [homeTeam.activity==teamAction(3)]
      GetBall -> Defend [order 2] : [homeTeam.activity==teamAction(2)]
      GetBall -> (junction 319) [order 1]
      (junction 320) -> GetBall
      (junction 321) -> GetBall
    (default) -> InPlay
  state [dist,ang] = calcBearing(goal) [function]
    (default) -> (junction 219) : % Calculate distance and angle to location
        | {
        | err = goal(1:2) - [position(1) position(2)];
        | dist = norm(err);
        | ang = angdiff(position(3),atan2(err(2),err(1)));
        | }
  state PlayerDistances [parallel]
    settings: executionOrder=2
    state FindObject [parallel]
      en,du:
      [objSeen,objDist,objAng] = detectObj(objects,obj);
      toObj = [objSeen,objDist,objAng];
      settings: executionOrder=1
  state [vel,done] = turnToPoint(goal) [function]
    note: Tracks a position. Once reached, the robot will turn in place until a reference angle is met.
    (default) -> (junction 255) : % Turn in place until the angular reference is met
        | {
        | done = false;
        | vel = [0;0;0];
        | [goalDist,goalAng] = calcBearing(goal(1:2));
        | }
    (junction 255) -> (junction 256) [order 1] : [goalAng > angThresh]
    (junction 255) -> (junction 257) [order 2]
    (junction 256) -> (junction 261) : {vel(3) = 1;}
    (junction 257) -> (junction 258) [order 1] : [goalAng < -angThresh]
    (junction 257) -> (junction 259) [order 2] : {done = true;}
    (junction 258) -> (junction 260) : {vel(3) = -1;}
    (junction 260) -> (junction 259)
    (junction 261) -> (junction 260)
  state vel = trackDetection(dist,ang) [function]
    note: Uses range and bearing to track an object
    (default) -> (junction 277) : {
        | vel = [0;0;0];
        | }
    (junction 277) -> (junction 276) [order 1] : % Turn in place
        | % if no detection
        | [dist < 0]
    (junction 276) -> (junction 286) : {vel(3) = 1;}
    (junction 277) -> (junction 278) [order 2]
    (junction 278) -> (junction 279) [order 1] : % Forward speed
        | [dist > distThresh]
    (junction 279) -> (junction 281) : {vel(1) = maxSpeed;}
    (junction 278) -> (junction 280) [order 2]
    (junction 281) -> (junction 280)
    (junction 280) -> (junction 282)
    (junction 282) -> (junction 283) [order 1] : % Turning speed
        | [ang > angThresh]
    (junction 283) -> (junction 289) : {vel(3) = maxTurnSpeed;}
    (junction 282) -> (junction 284) [order 2]
    (junction 284) -> (junction 285) [order 1] : [ang < -angThresh]
    (junction 284) -> (junction 287) [order 2]
    (junction 285) -> (junction 288) : {vel(3) = -1;}
    (junction 286) -> (junction 287)
    (junction 288) -> (junction 287)
    (junction 289) -> (junction 288)
  data: vel function_output; done function_output; goal function_input; goal function_input; dist function_output; ang function_output; goal function_input; vel function_output; done function_output; dist function_input; ang function_input; vel function_output; homeTeam input; position input; velocity input; nextVelocity output =[0;0;0]; players input; teammates input; objects input; objAng local; objDist local; objSeen local; angThresh parameter; distThresh parameter; maxSpeed parameter; maxTurnSpeed parameter; obj local =1; toObj output; robotIndex local =4
